simulink model "scheme_u2"  (R2023b)
settings: Solver=VariableStepAuto  StartTime=0.0  StopTime=20  RelTol=1e-3
values from neighbouring files (symbols this model uses):
  A = [-a_1 1; -a_0 0]    [init.m]
  A_0 = [-k_1 1; -k_0 0]    [init.m]
  b = [b_1; b_0]    [init.m]
  C = [1 0]    [init.m]
  k_0 = 4    [init.m]
  k_1 = 4    [init.m]
  theta = [k_0-a_0; k_1-a_1; b_0; b_1]    [init.m]
settings Model: Creator=lalayants  LastModifiedBy=lalayants

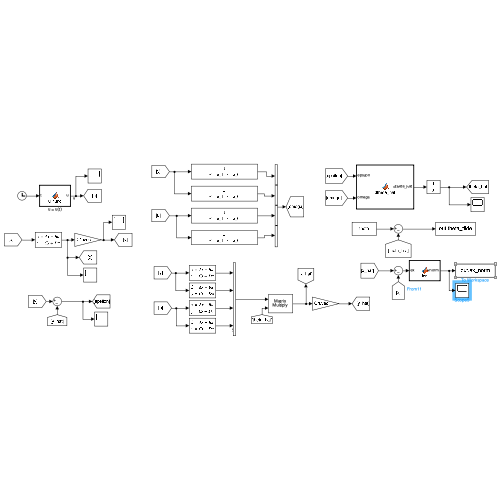
[thumbnail: Simulink's stored preview of the top-level diagram]
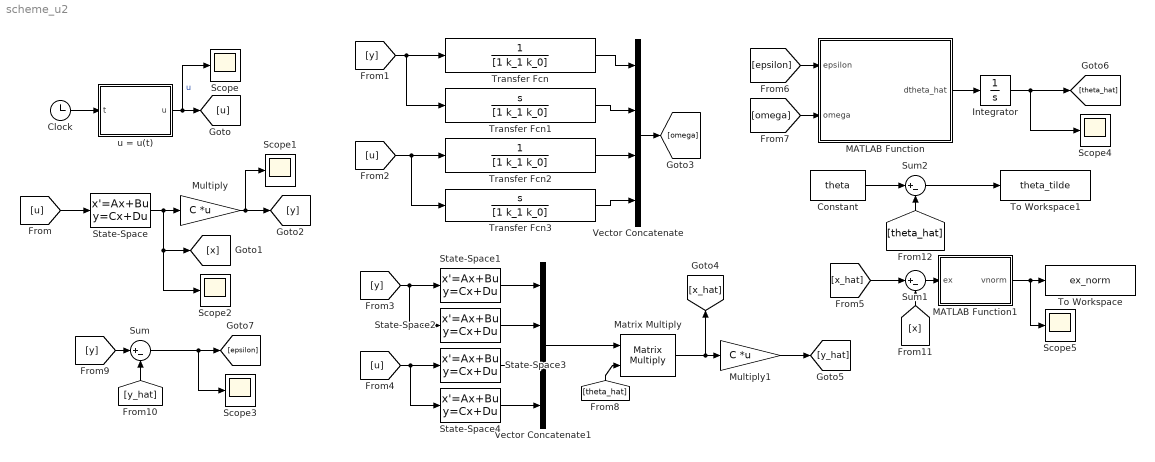
== system scheme_u2 ==
  Clock : Clock
  Constant : Constant  Value=theta
  Integrator : Integrator
  MATLAB Function : MATLAB Function  TreatAsAtomicUnit=on
  MATLAB Function1 : MATLAB Function  TreatAsAtomicUnit=on
  Matrix Multiply : Product  Multiplication=Matrix(*)
  Multiply : Gain  Gain=C  Multiplication=Matrix(K*u) (u vector)
  Multiply1 : Gain  Gain=C  Multiplication=Matrix(K*u) (u vector)
  Scope{,1..5} (6 alike) : Scope
  State-Space : StateSpace  A=A  B=b  C=eye(2)  D=[0; 0]  InitialCondition=0
  State-Space1 : StateSpace  A=A_0  B=[0; 1]  C=eye(2)  D=[0; 0]  InitialCondition=0
  State-Space2 : StateSpace  A=A_0  B=[1; 0]  C=eye(2)  D=[0; 0]  InitialCondition=0
  State-Space3 : StateSpace  A=A_0  B=[0; 1]  C=eye(2)  D=[0; 0]  InitialCondition=0
  State-Space4 : StateSpace  A=A_0  B=[1; 0]  C=eye(2)  D=[0; 0]  InitialCondition=0
  Sum : Sum  Inputs=|+-
  Sum1 : Sum  Inputs=|+-
  Sum2 : Sum  Inputs=|+-
  To Workspace : ToWorkspace  VariableName=ex_norm  SaveFormat=Timeseries  SampleTime=-1
  To Workspace1 : ToWorkspace  VariableName=theta_tilde  SaveFormat=Timeseries  SampleTime=-1
  Transfer Fcn : TransferFcn  Denominator=[1 k_1 k_0]
  Transfer Fcn1 : TransferFcn  Numerator=[1 0]  Denominator=[1 k_1 k_0]
  Transfer Fcn2 : TransferFcn  Denominator=[1 k_1 k_0]
  Transfer Fcn3 : TransferFcn  Numerator=[1 0]  Denominator=[1 k_1 k_0]
  Vector Concatenate : Concatenate  NumInputs=4
  Vector Concatenate1 : Concatenate  NumInputs=4  Mode=Multidimensional array  ConcatenateDimension=2
  u = u(t) : MATLAB Function  TreatAsAtomicUnit=on
  wires:
  Clock/1 -> u = u(t)/1(t)
  State-Space/1 -> [x], Scope2/1, Multiply/1
  u = u(t)/1(u) -> Scope/1, [u]  "u"
  [u] -> State-Space/1
  Multiply/1 -> Scope1/1, [y]
  [y] -> Transfer Fcn/1, Transfer Fcn1/1
  [u] -> Transfer Fcn3/1, Transfer Fcn2/1
  [y] -> State-Space2/1, State-Space1/1
  [u] -> State-Space4/1, State-Space3/1
  State-Space4/1 -> Vector Concatenate1/4
  State-Space3/1 -> Vector Concatenate1/3
  State-Space2/1 -> Vector Concatenate1/2
  State-Space1/1 -> Vector Concatenate1/1
  Transfer Fcn3/1 -> Vector Concatenate/4
  Transfer Fcn2/1 -> Vector Concatenate/3
  Transfer Fcn1/1 -> Vector Concatenate/2
  Transfer Fcn/1 -> Vector Concatenate/1
  Vector Concatenate/1 -> [omega]
  Multiply1/1 -> [y_hat]
  [epsilon] -> MATLAB Function/1(epsilon)
  [omega] -> MATLAB Function/2(omega)
  MATLAB Function/1(dtheta_hat) -> Integrator/1
  Integrator/1 -> [theta_hat], Scope4/1
  Matrix Multiply/1 -> [x_hat], Multiply1/1
  Vector Concatenate1/1 -> Matrix Multiply/1
  [theta_hat] -> Matrix Multiply/2
  [y] -> Sum/1
  [y_hat] -> Sum/2
  Sum/1 -> [epsilon], Scope3/1
  [x_hat] -> Sum1/1
  [x] -> Sum1/2
  Constant/1 -> Sum2/1
  Sum2/1 -> To Workspace1/1
  [theta_hat] -> Sum2/2
  Sum1/1 -> MATLAB Function1/1(ex)
  MATLAB Function1/1(vnorm) -> Scope5/1, To Workspace/1

== matlab function scheme_u2/MATLAB Function ==
  data: epsilon input; dtheta_hat output; omega input; gamma parameter
function dtheta_hat = dtheta_hat(epsilon, omega, gamma)

dtheta_hat = epsilon * omega * gamma;

== matlab function scheme_u2/u = u(t) ==
  data: t input; u output
function u = u_func(t)

u = 10 * sin(t) + 5 * cos(2*t) + 4 * cos(4*t) + 3 * cos(8*t);

== matlab function scheme_u2/MATLAB Function1 ==
  data: ex input; vnorm output
function vnorm = fcn(ex)

vnorm = norm(ex);
